simulink model "QNX_Node_Train_InOutProc"  (R2026a)
settings: Solver=VariableStepAuto
settings Model: DataDictionary=Architecture_DD.sldd  Creator=jaime  LastModifiedBy=jaime

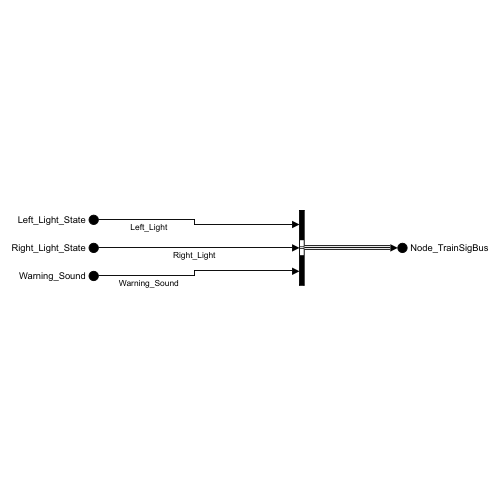
[thumbnail: Simulink's stored preview of the top-level diagram]
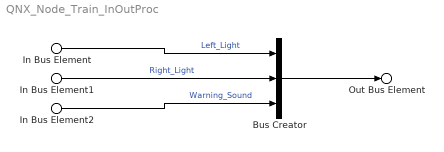
== system QNX_Node_Train_InOutProc ==
  In Bus Element : Inport  PortName=Left_Light_State
  In Bus Element1 : Inport  Port=2  PortName=Right_Light_State
  In Bus Element2 : Inport  Port=3  PortName=Warning_Sound
  Bus Creator : BusCreator  Inputs=3  OutDataTypeStr=Bus: Node_TrainSigBus
  Out Bus Element : Outport  PortName=Node_TrainSigBus
  wires:
  Bus Creator/1 -> Out Bus Element/1
  In Bus Element/1 -> Bus Creator/1  "Left_Light"
  In Bus Element1/1 -> Bus Creator/2  "Right_Light"
  In Bus Element2/1 -> Bus Creator/3  "Warning_Sound"
